simulink model "Pitch_Damper"  (Simulink 9.1)
settings: Solver=ode45  StartTime=0.0  StopTime=40.0  RelTol=1e-3  EnableMultiTasking=on
values from neighbouring files (symbols this model uses):
  D_act = [1 lambda]    [PitchDamp.m]    (also in PitchPilot.m)
  Den_sp = Den_sp(1:3)    [PitchPilot.m]
  Kcont = -0.063    [PitchDamp.m]
  Kq = 1    [PitchDamp.m]    (also in PitchPilot.m)
  N_act = Kact*lambda    [PitchDamp.m]    (also in PitchPilot.m)
  N_q_sp = N_q_sp(2:3)    [PitchPilot.m]
libraries: simulink x1
settings Model: Creator=MADIS03  LastModifiedBy=Andreas Surface Pro
settings DataIOCC: LimitDataPoints=on  SignalLoggingSaveFormat=ModelDataLogs
settings OptimizationCC: ExpressionDepthLimit=2147483647
settings DebuggingCC: SolverPrmCheckMsg=warning  FcnCallInpInsideContextMsg=warning  StateNameClashWarn=warning
settings HardwareCC: ProdBitPerPointer=64  ProdBitPerSizeT=64  ProdBitPerPtrDiffT=64  ProdLargestAtomicFloat=Float  ProdIntDivRoundTo=Zero  ProdEndianess=LittleEndian  ProdWordSize=64  ProdHWDeviceType=AMD->x86-64 (Windows64)
settings GRTTargetCC: GeneratePreprocessorConditionals=Disable all
settings ConfigComp: CovSFcnEnable=off

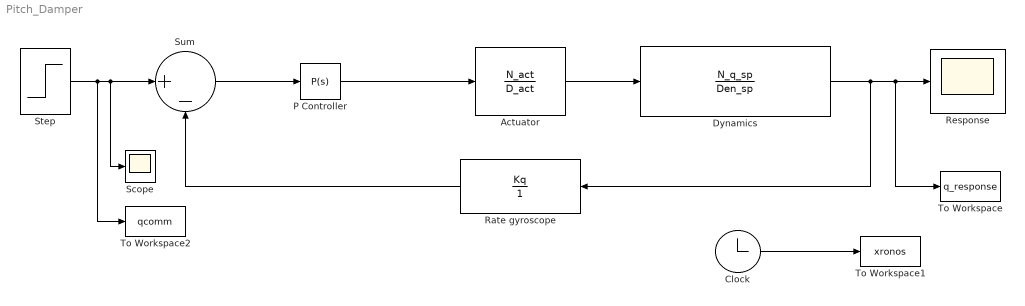
== system Pitch_Damper ==
  Actuator : TransferFcn  Numerator=N_act  Denominator=D_act
  Clock : Clock
  Dynamics : TransferFcn  Numerator=N_q_sp  Denominator=Den_sp
  P Controller : simulink/Continuous/PID Controller  Controller=P  TimeDomain=Continuous-time  SampleTime=-1  IntegratorMethod=Forward Euler  FilterMethod=Forward Euler  Form=Parallel  UseFilter=on  ControllerParametersSource=internal  P=Kcont  I=1  D=0  N=100  InitialConditionSource=internal  InitialConditionForIntegrator=0  InitialConditionForFilter=0  ExternalReset=none  LimitOutput=off  UpperSaturationLimit=inf  LowerSaturationLimit=-inf  LinearizeAsGain=on  AntiWindupMode=none  Kb=1  TrackingMode=off  Kt=1  PParamMin=[]  PParamMax=[]  IParamMin=[]  IParamMax=[]  DParamMin=[]  DParamMax=[]  NParamMin=[]  NParamMax=[]  KbParamMin=[]  KbParamMax=[]  KtParamMin=[]  KtParamMax=[]  POutMin=[]  POutMax=[]  IOutMin=[]  IOutMax=[]  DOutMin=[]  DOutMax=[]  NOutMin=[]  NOutMax=[]  KbOutMin=[]  KbOutMax=[]  KtOutMin=[]  KtOutMax=[]  IntegratorOutMin=[]  IntegratorOutMax=[]  FilterOutMin=[]  FilterOutMax=[]  SumOutMin=[]  SumOutMax=[]  SumI1OutMin=[]  SumI1OutMax=[]  SumI2OutMin=[]  SumI2OutMax=[]  SumI3OutMin=[]  SumI3OutMax=[]  SumDOutMin=[]  SumDOutMax=[]  SaturationOutMin=[]  SaturationOutMax=[]  IntegratorContinuousStateAttributes=''  IntegratorStateMustResolveToSignalObject=off  IntegratorRTWStateStorageClass=Auto  FilterContinuousStateAttributes=''  FilterStateMustResolveToSignalObject=off  FilterRTWStateStorageClass=Auto  DifferentiatorICPrevScaledInput=0  DifferentiatorOutMin=[]  DifferentiatorOutMax=[]  FilterDiffOutCoefMin=[]  FilterDiffOutCoefMax=[]  SumDenOutMin=[]  SumDenOutMax=[]  SumNumOutMin=[]  SumNumOutMax=[]  ReciprocalOutMin=[]  ReciprocalOutMax=[]  DivideOutMin=[]  DivideOutMax=[]  TunerSelectOption=Transfer Function Based (PID Tuner App)
  Rate gyroscope : TransferFcn  Numerator=Kq  Denominator=1
  Response : Scope
  Scope : Scope
  Step : Step  Time=0  SampleTime=0
  Sum : Sum  Inputs=|+-
  To Workspace : ToWorkspace  VariableName=q_response  SampleTime=-1
  To Workspace1 : ToWorkspace  VariableName=xronos  SampleTime=-1
  To Workspace2 : ToWorkspace  VariableName=qcomm  SampleTime=-1
      settings: Save2DSignal=2-D array (concatenate along first dimension)
  wires:
  Actuator/1 -> Dynamics/1
  Clock/1 -> To Workspace1/1
  Sum/1 -> P Controller/1
  P Controller/1 -> Actuator/1
  Dynamics/1 -> Rate gyroscope/1, Response/1, To Workspace/1
  Rate gyroscope/1 -> Sum/2
  Step/1 -> To Workspace2/1, Scope/1, Sum/1
